simulink model "ex10_planar_robot_ac"  (R2016b)
settings: Solver=ode3  StartTime=0.0  StopTime=10  FixedStep=0.001  MaxStep=0.001  RelTol=1e-3  EnableMultiTasking=on
values from neighbouring files (symbols this model uses):
  a1 = u_gen(15)    [classical_joint_planar_robot_simulink.m]    (also in ct_gravit_planar_robot_simulink.m = u_gen(13); ct_pid_planar_robot_simulink.m; ct_planar_robot_simulink.m = u_gen(13); ex_planar_robot_2dof.m = 1)
  a2 = u_gen(16)    [classical_joint_planar_robot_simulink.m]    (also in ct_gravit_planar_robot_simulink.m = u_gen(14); ct_pid_planar_robot_simulink.m; ct_planar_robot_simulink.m = u_gen(14); ex_planar_robot_2dof.m = 1)
  g = u_gen(17)    [classical_joint_planar_robot_simulink.m]    (also in ct_gravit_planar_robot_simulink.m; ct_pid_planar_robot_simulink.m; ct_planar_robot_simulink.m = u_gen(15); ex_planar_robot_2dof.m = 9.81)
  m1r = 0.8    [ex_planar_robot_2dof.m]
  m2r = 2.3    [ex_planar_robot_2dof.m]
settings Model: ExtModeTrigDuration=5000  Creator=Patrick  LastModifiedBy=kargto
settings SolverCC: PositivePriorityOrder=on
settings DataIOCC: LimitDataPoints=on  SaveFormat=Array
settings OptimizationCC: LifeSpan=inf
settings DebuggingCC: SolverPrmCheckMsg=warning  SFUnexpectedBacktrackingDiag=warning  SFNoUnconditionalDefaultTransitionDiag=warning  SFExecutionAtInitializationDiag=none
settings HardwareCC: ProdBitPerPointer=32  ProdBitPerSizeT=32  ProdBitPerPtrDiffT=32  ProdLargestAtomicFloat=None  ProdIntDivRoundTo=Undefined  ProdEndianess=Unspecified  ProdWordSize=32  ProdHWDeviceType=32-bit Generic
settings ModelReferenceCC: PropagateSignalLabelsOutOfModel=off
settings RTWCC: SystemTargetFile=quarc_win64.tlc  TemplateMakefile=quarc_default_tmf  Description=QUARC Win64 Target
settings STFCustomTargetCC: TargetPreCompLibLocation=C:\PROGRA~3\QUARC\lib\2014a\win64\release  ConcurrentExecutionCompliant=on  GeneratePreprocessorConditionals=Disable all  CombineOutputUpdateFcns=on  GRTInterface=off  SystemTargetFile=quarc_win64.tlc
settings GRTTargetCC: TargetPreCompLibLocation=C:\PROGRA~3\QUARC\lib\2014a\win64\release  TargetLangStandard=C89/C90 (ANSI)  ParMdlRefBuildCompliant=off  CompOptLevelCompliant=off  GeneratePreprocessorConditionals=Disable all  MatFileLogging=off  CPPClassGenCompliant=off  UseToolchainInfoCompliant=off  ExtMode=on  ExtModeMexFile=quarc_comm
settings ConfigComp: CovMetricSettings=dw  CovHtmlReporting=on  CovSaveCumulativeToWorkspaceVar=on  CovSaveSingleToWorkspaceVar=on  CovExternalEMLEnable=off  CovSFcnEnable=off

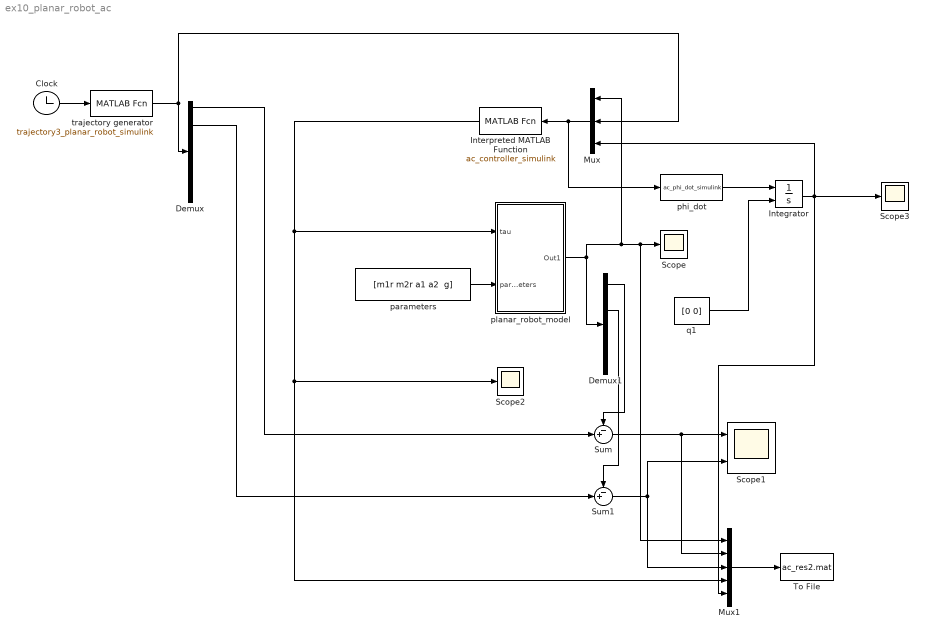
== system ex10_planar_robot_ac ==
  Clock : Clock
  Demux : Demux  Outputs=6
  Demux1 : Demux
  Integrator : Integrator  InitialConditionSource=external
  Interpreted MATLAB Function : MATLABFcn  MATLABFcn=ac_controller_simulink
  Mux : Mux  Inputs=3
  Mux1 : Mux  Inputs=5
  Scope : Scope
  Scope1 : Scope  NumInputPorts=2
  Scope2 : Scope
  Scope3 : Scope
  Sum : Sum  Inputs=-+|
  Sum1 : Sum  Inputs=-+|
  To File : ToFile  Filename=ac_res2.mat  MatrixName=ac
  parameters : Constant  Value="[m1r m2r a1 a2  g]"
  phi_dot : MATLABFcn  MATLABFcn=ac_phi_dot_simulink
  planar_robot_model : Subsystem
  q1 : Constant  Value=[0 0]
  trajectory generator : MATLABFcn  MATLABFcn=trajectory3_planar_robot_simulink
  wires:
  Mux/1 -> phi_dot/1, Interpreted MATLAB Function/1
  Clock/1 -> trajectory generator/1
  trajectory generator/1 -> Demux/1, Mux/2
  Demux/1 -> Sum/2
  Demux1/1 -> Sum/1
  Sum/1 -> Mux1/2, Scope1/1
  Sum1/1 -> Scope1/2, Mux1/3
  Demux1/2 -> Sum1/1
  Demux/2 -> Sum1/2
  Interpreted MATLAB Function/1 -> Mux1/4, Scope2/1, planar_robot_model/1(tau)
  Mux1/1 -> To File/1
  phi_dot/1 -> Integrator/1
  q1/1 -> Integrator/2
  Integrator/1 -> Mux1/5, Scope3/1, Mux/3
  planar_robot_model/1(Out1) -> Demux1/1, Mux/1, Mux1/1, Scope/1
  parameters/1 -> planar_robot_model/2(parameters)

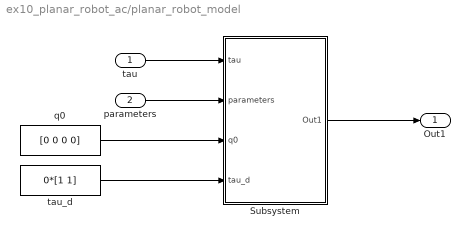
== system ex10_planar_robot_ac/planar_robot_model ==
  tau : Inport
  parameters : Inport  Port=2
  Subsystem : Subsystem
  q0 : Constant  Value=[0 0 0 0]
  tau_d : Constant  Value=0*[1 1]
  Out1 : Outport
  wires:
  Subsystem/1(Out1) -> Out1/1
  q0/1 -> Subsystem/3(q0)
  tau_d/1 -> Subsystem/4(tau_d)
  tau/1 -> Subsystem/1(tau)
  parameters/1 -> Subsystem/2(parameters)

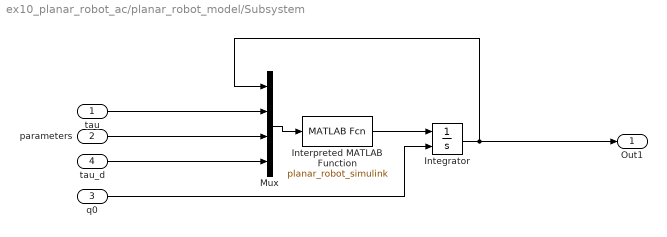
== system ex10_planar_robot_ac/planar_robot_model/Subsystem ==
  tau : Inport
  parameters : Inport  Port=2
  q0 : Inport  Port=3
  tau_d : Inport  Port=4
  Integrator : Integrator  InitialConditionSource=external
  Interpreted MATLAB Function : MATLABFcn  MATLABFcn=planar_robot_simulink  OutputDimensions=4
  Mux : Mux
  Out1 : Outport
  wires:
  Interpreted MATLAB Function/1 -> Integrator/1
  q0/1 -> Integrator/2
  Mux/1 -> Interpreted MATLAB Function/1
  Integrator/1 -> Out1/1, Mux/1
  tau/1 -> Mux/2
  parameters/1 -> Mux/3
  tau_d/1 -> Mux/4
